simulink model "TEST_IPM_2_0"  (R2019b)
settings: configuration reference "Configuration" (kept outside this file)
PreLoadFcn:
  | RTWConfigurationCB('preloadfcn', bdroot);
values from neighbouring files (symbols this model uses):
  MParamFbase = 200.0    [TEST_IPM_LIB.sldd]
  MParamIbase = 360.0    [TEST_IPM_LIB.sldd]
  MParamLd = 8.0E-5    [TEST_IPM_LIB.sldd]
  MParamLq = 0.00028    [TEST_IPM_LIB.sldd]
  MParamRs = 0.014    [TEST_IPM_LIB.sldd]
  PWM_TPBRD_HALF = 5000.0    [TEST_IPM_LIB.sldd]
  Ts_10kHz = 0.0001    [TEST_IPM_LIB.sldd]
  Ts_1kHz = 0.001    [TEST_IPM_LIB.sldd]
undefined symbols (not defined in the file or in its folder): DiscIntNeverNeededParam, Down, GPTRIP1SEL, GPTRIP2SEL, TZ1, TZ2, Up
libraries: c280xlib x24, c2837xDlib x18, dsparch4 x11, c2802xlib x10, powerlib_meascontrol x9, dspstat3 x2, c2000lib x1, c2806xlib x1, idelinklib_common x1
(part 3 of 6)

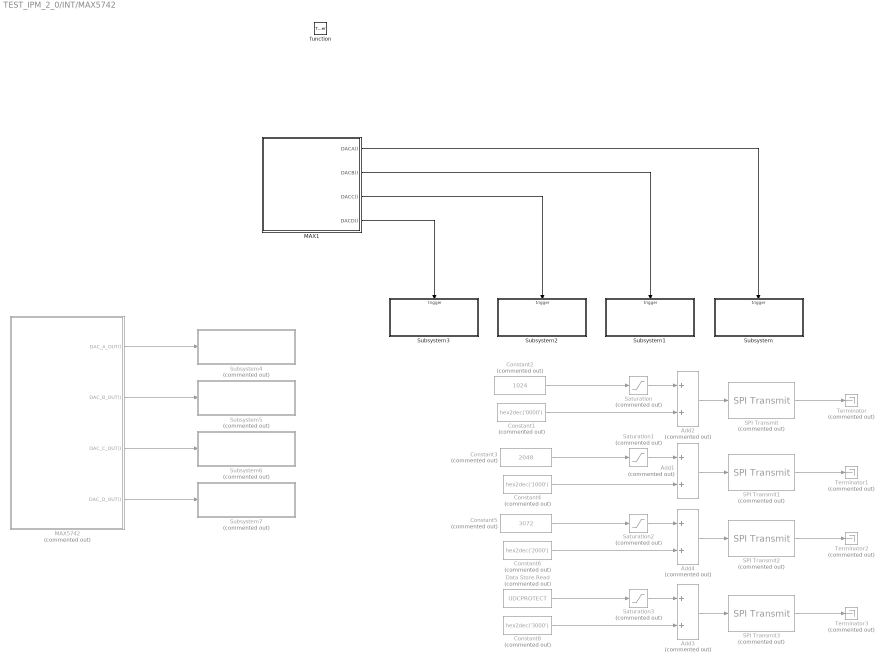
== system TEST_IPM_2_0/INT/MAX5742 ==
  function : TriggerPort  TriggerType=function-call  VariantControl=Variant
  Add{1..4} (4 alike) : Sum  Commented=on
  Constant1 : Constant  Commented=on  Value=hex2dec('0000')  OutDataTypeStr=uint16  SampleTime=-1
  Constant2 : Constant  Priority=102  Commented=on  Value=1024  OutDataTypeStr=Inherit: Inherit via back propagation  SampleTime=-1
  Constant3 : Constant  Priority=107  Commented=on  Value=2048  OutDataTypeStr=Inherit: Inherit via back propagation  SampleTime=-1
  Constant4 : Constant  Commented=on  Value=hex2dec('1000')  OutDataTypeStr=uint16  SampleTime=-1
  Constant5 : Constant  Priority=112  Commented=on  Value=3072  OutDataTypeStr=Inherit: Inherit via back propagation  SampleTime=-1
  Constant6 : Constant  Commented=on  Value=hex2dec('2000')  OutDataTypeStr=uint16  SampleTime=-1
  Constant8 : Constant  Commented=on  Value=hex2dec('3000')  OutDataTypeStr=uint16  SampleTime=-1
  Data Store Read : DataStoreRead  Commented=on  DataStoreName=UDCPROTECT
  MAX1 : MATLAB Function  TreatAsAtomicUnit=on
  MAX5742 : Stateflow chart  Commented=on  BlockKeywords=__PRM__SERIALIZED__DATA__:Stateflow Chart,Stateflow Diagram  TreatAsAtomicUnit=on
  SPI Transmit : c280xlib/SPI Transmit  Commented=on  SPISelect=SPI_B  ClockPolarity=Falling_edge  ClockPhase=No_delay  SPIModule=uint32(0)  Mode=Master  BusSpeed=uint32(1000000)  FirstBitToTransfer=Most significant bit (MSB)  ClockMode=0  BlockFunction=Write  EnableRegisterAddress=on  RegisterAddress=0  OutputDataType=int8  OutputDataLength=1  BlockingMode=off  DataBits=16  UseCustomSSPin=Provided by the SPI peripheral  ActiveLowSSPin=Active low  Pin=0
      settings: SourceProductName=Embedded Coder Support Package for Texas Instruments C2000 Processors  SourceProductBaseCode=TIC2000
  SPI Transmit1 : c280xlib/SPI Transmit  Commented=on  SPISelect=SPI_B  ClockPolarity=Rising_edge  ClockPhase=No_delay  SPIModule=uint32(0)  Mode=Master  BusSpeed=uint32(1000000)  FirstBitToTransfer=Most significant bit (MSB)  ClockMode=0  BlockFunction=Write  EnableRegisterAddress=on  RegisterAddress=0  OutputDataType=int8  OutputDataLength=1  BlockingMode=off  DataBits=16  UseCustomSSPin=Provided by the SPI peripheral  ActiveLowSSPin=Active low  Pin=0
      settings: SourceProductName=Embedded Coder Support Package for Texas Instruments C2000 Processors  SourceProductBaseCode=TIC2000
  SPI Transmit2 : c280xlib/SPI Transmit  Commented=on  SPISelect=SPI_B  ClockPolarity=Rising_edge  ClockPhase=No_delay  SPIModule=uint32(0)  Mode=Master  BusSpeed=uint32(1000000)  FirstBitToTransfer=Most significant bit (MSB)  ClockMode=0  BlockFunction=Write  EnableRegisterAddress=on  RegisterAddress=0  OutputDataType=int8  OutputDataLength=1  BlockingMode=off  DataBits=16  UseCustomSSPin=Provided by the SPI peripheral  ActiveLowSSPin=Active low  Pin=0
      settings: SourceProductName=Embedded Coder Support Package for Texas Instruments C2000 Processors  SourceProductBaseCode=TIC2000
  SPI Transmit3 : c280xlib/SPI Transmit  Commented=on  SPISelect=SPI_B  ClockPolarity=Rising_edge  ClockPhase=No_delay  SPIModule=uint32(0)  Mode=Master  BusSpeed=uint32(1000000)  FirstBitToTransfer=Most significant bit (MSB)  ClockMode=0  BlockFunction=Write  EnableRegisterAddress=on  RegisterAddress=0  OutputDataType=int8  OutputDataLength=1  BlockingMode=off  DataBits=16  UseCustomSSPin=Provided by the SPI peripheral  ActiveLowSSPin=Active low  Pin=0
      settings: SourceProductName=Embedded Coder Support Package for Texas Instruments C2000 Processors  SourceProductBaseCode=TIC2000
  Saturation{,1..3} (4 alike) : Saturate  Commented=on  UpperLimit=4095  LowerLimit=0  OutDataTypeStr=uint16
  Subsystem : Subsystem
  Subsystem1 : Subsystem
  Subsystem2 : Subsystem
  Subsystem3 : Subsystem
  Subsystem4 : Subsystem  Commented=on
  Subsystem5 : Subsystem  Commented=on
  Subsystem6 : Subsystem  Commented=on
  Subsystem7 : Subsystem  Commented=on
  Terminator{,1..3} (4 alike) : Terminator  Commented=on
  wires:
  MAX1/4(DACD()) -> Subsystem3/Trigger
  MAX1/3(DACC()) -> Subsystem2/Trigger
  MAX1/2(DACB()) -> Subsystem1/Trigger
  MAX1/1(DACA()) -> Subsystem/Trigger
  SPI Transmit/1 -> Terminator/1
  Add2/1 -> SPI Transmit/1
  Saturation/1 -> Add2/1
  Constant2/1 -> Saturation/1
  Constant1/1 -> Add2/2
  SPI Transmit1/1 -> Terminator1/1
  Constant4/1 -> Add1/2
  Add1/1 -> SPI Transmit1/1
  Saturation1/1 -> Add1/1
  Constant3/1 -> Saturation1/1
  Constant5/1 -> Saturation2/1
  Constant6/1 -> Add4/2
  Add4/1 -> SPI Transmit2/1
  Saturation2/1 -> Add4/1
  SPI Transmit2/1 -> Terminator2/1
  Saturation3/1 -> Add3/1
  Add3/1 -> SPI Transmit3/1
  SPI Transmit3/1 -> Terminator3/1
  Constant8/1 -> Add3/2
  Data Store Read/1 -> Saturation3/1
  MAX5742/1(DAC_A_OUT()) -> Subsystem4/Trigger
  MAX5742/2(DAC_B_OUT()) -> Subsystem5/Trigger
  MAX5742/3(DAC_C_OUT()) -> Subsystem6/Trigger
  MAX5742/4(DAC_D_OUT()) -> Subsystem7/Trigger

== system TEST_IPM_2_0/INT/Motor Control ==
  function : TriggerPort  TriggerType=function-call  VariantControl=Variant
  Adjusting Mode : Subsystem  TreatAsAtomicUnit=on
  Clark Transformation : Subsystem
  Current_PI : Subsystem  TreatAsAtomicUnit=on
      settings: RTWSystemCode=Inline
  Data Store Read1 : DataStoreRead  DataStoreName=ControlAng
  Data Store Read13 : DataStoreRead  DataStoreName=ControlAng
  Data Store Read14 : DataStoreRead  DataStoreName=Ud_in
  Data Store Read15 : DataStoreRead  DataStoreName=Uq_in
  Data Store Read16 : DataStoreRead  DataStoreName=W_Current
  Data Store Read2 : DataStoreRead  DataStoreName=ControlMode
  Data Store Read5 : DataStoreRead  DataStoreName=U_Current
  Data Store Read6 : DataStoreRead  DataStoreName=V_Current
  Data Store Write : DataStoreWrite  DataStoreName=COMPARE_A
  Data Store Write1 : DataStoreWrite  DataStoreName=COMPARE_B
  Data Store Write2 : DataStoreWrite  DataStoreName=COMPARE_C
  Data Store Write6 : DataStoreWrite  DataStoreName=Iq_FBK
  Data Store Write8 : DataStoreWrite  DataStoreName=Id_FBK
  Demux : Demux  Outputs=3
  Error : Subsystem  TreatAsAtomicUnit=on
  FbLMode : Subsystem  TreatAsAtomicUnit=on
  IF : Subsystem  TreatAsAtomicUnit=on
  Park Transformation : Subsystem
  SVPWM : Subsystem  TreatAsAtomicUnit=on
      settings: RTWSystemCode=Inline
  SpeedMode : Subsystem  TreatAsAtomicUnit=on
  "Stop " : Subsystem  TreatAsAtomicUnit=on
  Switch Case : SwitchCase  CaseConditions={0,1,2,3,4,5,6}
  TorqueMode : Subsystem  TreatAsAtomicUnit=on
  VF : Subsystem  TreatAsAtomicUnit=on
  wires:
  Data Store Read2/1 -> Switch Case/1
  Switch Case/1 -> Adjusting Mode/Action
  Switch Case/6 -> "Stop "/Action
  Switch Case/8 -> Error/Action
  Switch Case/2 -> VF/Action
  Switch Case/3 -> IF/Action
  Switch Case/4 -> TorqueMode/Action
  Switch Case/5 -> SpeedMode/Action
  Data Store Read1/1 -> SVPWM/3(Angle)
  Current_PI/1(Ud_Reference) -> SVPWM/1(Ud_Reference)
  Current_PI/2(Uq_Reference) -> SVPWM/2(Uq_Reference)
  SVPWM/1(COMPARE) -> Demux/1
  Demux/1 -> Data Store Write/1
  Demux/2 -> Data Store Write1/1
  Demux/3 -> Data Store Write2/1
  Data Store Read14/1 -> Current_PI/1(Ud)
  Data Store Read15/1 -> Current_PI/2(Uq)
  Switch Case/7 -> FbLMode/Action
  Data Store Read6/1 -> Clark Transformation/2(V)
  Data Store Read13/1 -> Park Transformation/3(theta)
  Clark Transformation/1(Alpha) -> Park Transformation/1(Alpha)
  Data Store Read16/1 -> Clark Transformation/3(W)
  Data Store Read5/1 -> Clark Transformation/1(U)
  Park Transformation/2(Q) -> Data Store Write6/1
  Park Transformation/1(D) -> Data Store Write8/1
  Clark Transformation/2(Beta) -> Park Transformation/2(Beta)

== system TEST_IPM_2_0/INT/Read Rotor Position ==
  function : TriggerPort  TriggerType=function-call  VariantControl=Variant
  Data Store Read : DataStoreRead  Priority=3  DataStoreName=SPIC_Tx
  Data Store Read1 : DataStoreRead  Priority=5  DataStoreName=SPIC_Tx
  Data Store Read3 : DataStoreRead  DataStoreName=ResloverMid
  Data Store Write : DataStoreWrite  DataStoreName=ResloverAng
  Data Store Write1 : DataStoreWrite  DataStoreName=SPIC_Rx
  Data Store Write14 : DataStoreWrite  DataStoreName=THERMAL_N
  Data Store Write2 : DataStoreWrite  DataStoreName=N_FBK
  Data Store Write3 : DataStoreWrite  DataStoreName=ResloverFaultRead
  Digital Output1 : c2837xDlib/Digital Output  GPIO_Number=GPIO48~GPIO55  GPIO_Bit0=off  GPIO_BIT0_Toggle=off  GPIO_Bit1=off  GPIO_BIT1_Toggle=off  GPIO_Bit2=off  GPIO_BIT2_Toggle=off  GPIO_Bit3=off  GPIO_BIT3_Toggle=off  GPIO_Bit4=off  GPIO_BIT4_Toggle=off  GPIO_Bit5=on  GPIO_BIT5_Toggle=off  GPIO_Bit6=off  GPIO_BIT6_Toggle=off  GPIO_Bit7=off  GPIO_BIT7_Toggle=off
      settings: SourceProductName=Embedded Coder Support Package for Texas Instruments C2000 Processors  SourceProductBaseCode=TIC2000
  Digital Output2 : c2837xDlib/Digital Output  GPIO_Number=GPIO48~GPIO55  GPIO_Bit0=off  GPIO_BIT0_Toggle=off  GPIO_Bit1=off  GPIO_BIT1_Toggle=off  GPIO_Bit2=off  GPIO_BIT2_Toggle=off  GPIO_Bit3=off  GPIO_BIT3_Toggle=off  GPIO_Bit4=off  GPIO_BIT4_Toggle=off  GPIO_Bit5=off  GPIO_BIT5_Toggle=off  GPIO_Bit6=on  GPIO_BIT6_Toggle=off  GPIO_Bit7=off  GPIO_BIT7_Toggle=off
      settings: SourceProductName=Embedded Coder Support Package for Texas Instruments C2000 Processors  SourceProductBaseCode=TIC2000
  Gain : Gain  Gain=2*pi
  MATLAB Function : MATLAB Function  TreatAsAtomicUnit=on
  "RAW_DATA2Angle " : MATLAB Function  TreatAsAtomicUnit=on
  ResloverWR1 : Constant  Priority=6  OutDataTypeStr=Inherit: Inherit via back propagation  SampleTime=-1
  ResloverWR2 : Constant  Priority=6  OutDataTypeStr=Inherit: Inherit via back propagation  SampleTime=-1
  SPI Master Transfer : c280xlib/SPI Master Transfer  SPISelect=SPI_C  ClockPolarity=Rising_edge  ClockPhase=No_delay  SPIModule=uint32(0)  Mode=Master  BusSpeed=uint32(1000000)  FirstBitToTransfer=Most significant bit (MSB)  ClockMode=0  BlockFunction=Transfer  EnableRegisterAddress=off  RegisterAddress=0  OutputDataType=int8  OutputDataLength=1  DataBits=16  UseCustomSSPin=Provided by the SPI peripheral  ActiveLowSSPin=Active low  Pin=1
      settings: SourceProductName=Embedded Coder Support Package for Texas Instruments C2000 Processors  SourceProductBaseCode=TIC2000
  SPI Master Transfer1 : c280xlib/SPI Master Transfer  SPISelect=SPI_C  ClockPolarity=Rising_edge  ClockPhase=No_delay  SPIModule=uint32(0)  Mode=Master  BusSpeed=uint32(1000000)  FirstBitToTransfer=Most significant bit (MSB)  ClockMode=0  BlockFunction=Transfer  EnableRegisterAddress=off  RegisterAddress=0  OutputDataType=int8  OutputDataLength=1  DataBits=8  UseCustomSSPin=Provided by the SPI peripheral  ActiveLowSSPin=Active low  Pin=1
      settings: SourceProductName=Embedded Coder Support Package for Texas Instruments C2000 Processors  SourceProductBaseCode=TIC2000
  SpeedCal : Subsystem  TreatAsAtomicUnit=on
  wires:
  Data Store Read/1 -> SPI Master Transfer/1
  SPI Master Transfer/1 -> "RAW_DATA2Angle "/1(Raw_Data), Data Store Write1/1
  ResloverWR1/1 -> Digital Output1/1
  Data Store Read3/1 -> "RAW_DATA2Angle "/2(Mid_Position)
  "RAW_DATA2Angle "/1(Angle_out) -> Gain/1
  SpeedCal/1(Out1) -> Data Store Write14/1, Data Store Write2/1
  MATLAB Function/1(FunCall()) -> SpeedCal/Trigger
  Data Store Read1/1 -> SPI Master Transfer1/1
  SPI Master Transfer1/1 -> Data Store Write3/1
  ResloverWR2/1 -> Digital Output2/1
  Gain/1 -> SpeedCal/1(In1), Data Store Write/1

== system TEST_IPM_2_0/INT/ePWM ==
  function : TriggerPort  TriggerType=function-call  VariantControl=Variant
  Constant2 : Constant  Value=[0 0]  OutDataTypeStr=uint16  SampleTime=-1
  Constant3 : Constant  Value=[1 2]  OutDataTypeStr=uint16  SampleTime=-1
  Data Store Read1 : DataStoreRead  DataStoreName=STOP
  Data Store Read3 : DataStoreRead  DataStoreName=COMPARE_A
  Data Store Read4 : DataStoreRead  DataStoreName=COMPARE_B
  Data Store Read7 : DataStoreRead  DataStoreName=COMPARE_C
  Demux : Demux  Outputs=2
  If : If  IfExpression=u1 == 1
  If Action Subsystem : Subsystem  TreatAsAtomicUnit=on
  Switch : Switch  Criteria=u2 ~= 0
  ePWM : c2802xlib/ePWM  useModule=ePWM1  ePWMxLINKTBPRD=Not Linked  periodUnits=Clock cycles  timerSource=Specify via dialog  timerPeriod_clk=PWM_TPBRD  timerPeriod_sec=Tsw  tbshadow=Counter equals to zero  countingMode=Up-Down  phaseActiveEnable=Disable  phaseDirection=Count down after sync  phaseActive=0  synchronizationEnable=off  dcaevt1Sync=off  dcbevt1Sync=off  synchronizationOption=Counter equals to zero (CTR=Zero)  clockPrescale=1  HSclockPrescale=1  enswap=off  ePWMxAStatus=on  ePWMxAactionLogic1=Do nothing  ePWMxAactionLogic2=Do nothing  ePWMxAactionLogic3=Clear  ePWMxAactionLogic4=Set  ePWMxAactionLogic5=Do nothing  ePWMxAactionLogic6=Do nothing  ePWMxALoadMode=Load on counter equals to zero (CTR=Zero)  ePWMxACSFenable=on  ePWMxACSFvalue=Forcing disable  ePWMxASFreload=Immediate  ePWMxBStatus=on  ePWMxBactionLogic1=Do nothing  ePWMxBactionLogic2=Do nothing  ePWMxBactionLogic3=Clear  ePWMxBactionLogic4=Set  ePWMxBactionLogic5=Do nothing  ePWMxBactionLogic6=Do nothing  ePWMxBLoadMode=Load on counter equals to zero (CTR=Zero)  ePWMxBCSFenable=on  ePWMxBCSFvalue=Forcing disable  ePWMxBSFreload=Immediate  ePWNxBOutWay=off  ePWMxLINKCMPA=Not Linked  CMPAUnits=Clock cycles  CMPASource=Input port  CMPAValue_per=50  CMPAValue_clk=PWM_TPBRD_HALF  enCMPAshadow=Counter equals to zero  ePWMxLINKCMPB=Not Linked  CMPBUnits=Percentages  CMPBSource=Specify via dialog  CMPBValue_per=50  CMPBValue_clk=32000  enCMPBshadow=Counter equals to zero  ePWMxLINKCMPC=Not Linked  CMPCUnits=Clock cycles  CMPCSource=Specify via dialog  CMPCValue_per=50  CMPCValue_clk=32000  enCMPCshadow=Counter equals to zero  ePWMxLINKCMPD=Not Linked  CMPDUnits=Clock cycles  CMPDSource=Specify via dialog  CMPDValue_per=50  CMPDValue_clk=32000  enCMPDshadow=Counter equals to zero  enableDBePWMxA=on  enableDBePWMxB=on  enhalfcycle=off  DBpolarity=Active high complementary (AHC)  DBedgeDelay=Positive  DBSource_ePWMxA=ePWMxA  DBSource_ePWMxB=ePWMxB  DBperiodSource=Specify via dialog  REDperiod=PWM_TDEAD  FEDperiod=PWM_TDEAD  adcstartModuleA=on  adcrequestEventA=First event  adcstartEventA=Digital Compare Module A Event 1 start of conversion (DCAEVT1.soc)  adcstartEventA_type2=Counter equals to zero (CTR=Zero)  adcstartModuleB=off  adcrequestEventB=First event  adcstartEventB=Counter equals to zero (CTR=Zero)  adcstartEventB_type2=Counter equals to zero (CTR=Zero)  intEn=off  intPrd=First event  intSel=Counter equals to zero (CTR=Zero)  intSel_type2=Counter equals to period (CTR=PRD)  hrpe=off  enHRPWM=off  HRPWM_LoadMode=Counter equals to period (CTR=PRD)  HRPWM_CTLMode=Duty or Period control mode  HRPWM_EDGMode=Both edge  hrpeb=off  enHRPWMB=off  HRPWM_LoadModeB=Counter equals to zero (CTR=ZERO)  HRPWM_CTLModeB=Duty or Period control mode  HRPWM_EDGModeB=Both edge  enSFO=on  enautoconv=on  chopperEnable=off  chopperFrequency=1  chopperFirstwidth=1  chopperDuty=12.5%  tripZonesource=Specify via dialog  tzselOSHT1=off  tzselOSHT2=off  tzselOSHT3=off  tzselOSHDCAEV1=off  tzselOSHDCBEV1=off  tzselCBC1=off  tzselCBC2=off  tzselCBC3=off  tzselCBCDCAEV2=off  tzselCBCDCBEV2=off  tzselOSHT4=off  tzselOSHT5=off  tzselOSHT6=off  tzselCBC4=off  tzselCBC5=off  tzselCBC6=off  enTzOstIntr=on  enTzCbcIntr=off  enTzDCAEVT1Intr=off  enTzDCAEVT2Intr=off  enTzDCBEVT1Intr=off  enTzDCBEVT2Intr=off  ePWMxAforced=Low  ePWMxBforced=Low  DCAEVT1forced=No action  DCBEVT1forced=No action  DCAEVT2forced=No action  DCBEVT2forced=No action  dcah=Trip Zone 1 input (TZ1)  dcal=Trip Zone 2 input (TZ2)  dcbh=Trip Zone 1 input (TZ1)  dcbl=Trip Zone 2 input (TZ2)  dcah_type2=GPTRIP1SEL/(TZ1)  dcal_type2=GPTRIP2SEL/(TZ2)  dcbh_type2=GPTRIP1SEL/(TZ1)  dcbl_type2=GPTRIP2SEL/(TZ2)  gendcaevt1=Event disabled  gendcaevt2=Event disabled  gendcbevt1=Event disabled  gendcbevt2=Event disabled  dcaevt1src=DCAEVT1 with sync  dcaevt2src=DCAEVT2 with sync  dcbevt1src=DCBEVT1 with sync  dcbevt2src=DCBEVT2 with sync  pulsesel=Counter equals to zero (CTR=Zero)  blankinv=off  blankoffset=0  blankwidth=0  evsrcsel=Filtered version of DCAEVT1 (DCAEVT1FILT)  encape=off  PwmType=C2000_Type4
      settings: SourceProductName=Embedded Coder Support Package for Texas Instruments C2000 Processors
  ePWM1 : c2802xlib/ePWM  useModule=ePWM2  ePWMxLINKTBPRD=Not Linked  periodUnits=Clock cycles  timerSource=Specify via dialog  timerPeriod_clk=PWM_TPBRD  timerPeriod_sec=Tsw  tbshadow=Counter equals to zero  countingMode=Up-Down  phaseActiveEnable=Set counter to phase value specified via dialog  phaseDirection=Count down after sync  phaseActive=0  synchronizationEnable=off  dcaevt1Sync=off  dcbevt1Sync=off  synchronizationOption=Disable  clockPrescale=1  HSclockPrescale=1  enswap=off  ePWMxAStatus=on  ePWMxAactionLogic1=Do nothing  ePWMxAactionLogic2=Do nothing  ePWMxAactionLogic3=Clear  ePWMxAactionLogic4=Set  ePWMxAactionLogic5=Do nothing  ePWMxAactionLogic6=Do nothing  ePWMxALoadMode=Load on counter equals to zero (CTR=Zero)  ePWMxACSFenable=on  ePWMxACSFvalue=Forcing disable  ePWMxASFreload=Immediate  ePWMxBStatus=on  ePWMxBactionLogic1=Do nothing  ePWMxBactionLogic2=Do nothing  ePWMxBactionLogic3=Clear  ePWMxBactionLogic4=Set  ePWMxBactionLogic5=Do nothing  ePWMxBactionLogic6=Do nothing  ePWMxBLoadMode=Load on counter equals to zero (CTR=Zero)  ePWMxBCSFenable=on  ePWMxBCSFvalue=Forcing disable  ePWMxBSFreload=Immediate  ePWNxBOutWay=off  ePWMxLINKCMPA=Not Linked  CMPAUnits=Clock cycles  CMPASource=Input port  CMPAValue_per=50  CMPAValue_clk=PWM_TPBRD_HALF  enCMPAshadow=Counter equals to zero  ePWMxLINKCMPB=Not Linked  CMPBUnits=Percentages  CMPBSource=Specify via dialog  CMPBValue_per=50  CMPBValue_clk=32000  enCMPBshadow=Counter equals to zero  ePWMxLINKCMPC=Not Linked  CMPCUnits=Clock cycles  CMPCSource=Specify via dialog  CMPCValue_per=50  CMPCValue_clk=32000  enCMPCshadow=Counter equals to zero  ePWMxLINKCMPD=Not Linked  CMPDUnits=Clock cycles  CMPDSource=Specify via dialog  CMPDValue_per=50  CMPDValue_clk=32000  enCMPDshadow=Counter equals to zero  enableDBePWMxA=on  enableDBePWMxB=on  enhalfcycle=off  DBpolarity=Active high complementary (AHC)  DBedgeDelay=Positive  DBSource_ePWMxA=ePWMxA  DBSource_ePWMxB=ePWMxB  DBperiodSource=Specify via dialog  REDperiod=PWM_TDEAD  FEDperiod=PWM_TDEAD  adcstartModuleA=off  adcrequestEventA=First event  adcstartEventA=Digital Compare Module A Event 1 start of conversion (DCAEVT1.soc)  adcstartEventA_type2=Counter equals to period (CTR=PRD)  adcstartModuleB=off  adcrequestEventB=First event  adcstartEventB=Counter equals to zero (CTR=Zero)  adcstartEventB_type2=Counter equals to zero (CTR=Zero)  intEn=off  intPrd=First event  intSel=Counter equals to zero (CTR=Zero)  intSel_type2=Counter equals to period (CTR=PRD)  hrpe=off  enHRPWM=off  HRPWM_LoadMode=Counter equals to period (CTR=PRD)  HRPWM_CTLMode=Duty or Period control mode  HRPWM_EDGMode=Both edge  hrpeb=off  enHRPWMB=off  HRPWM_LoadModeB=Counter equals to zero (CTR=ZERO)  HRPWM_CTLModeB=Duty or Period control mode  HRPWM_EDGModeB=Both edge  enSFO=on  enautoconv=on  chopperEnable=off  chopperFrequency=1  chopperFirstwidth=1  chopperDuty=12.5%  tripZonesource=Specify via dialog  tzselOSHT1=off  tzselOSHT2=off  tzselOSHT3=off  tzselOSHDCAEV1=off  tzselOSHDCBEV1=off  tzselCBC1=off  tzselCBC2=off  tzselCBC3=off  tzselCBCDCAEV2=off  tzselCBCDCBEV2=off  tzselOSHT4=off  tzselOSHT5=off  tzselOSHT6=off  tzselCBC4=off  tzselCBC5=off  tzselCBC6=off  enTzOstIntr=on  enTzCbcIntr=off  enTzDCAEVT1Intr=off  enTzDCAEVT2Intr=off  enTzDCBEVT1Intr=off  enTzDCBEVT2Intr=off  ePWMxAforced=Low  ePWMxBforced=Low  DCAEVT1forced=No action  DCBEVT1forced=No action  DCAEVT2forced=No action  DCBEVT2forced=No action  dcah=Trip Zone 1 input (TZ1)  dcal=Trip Zone 2 input (TZ2)  dcbh=Trip Zone 1 input (TZ1)  dcbl=Trip Zone 2 input (TZ2)  dcah_type2=GPTRIP1SEL/(TZ1)  dcal_type2=GPTRIP2SEL/(TZ2)  dcbh_type2=GPTRIP1SEL/(TZ1)  dcbl_type2=GPTRIP2SEL/(TZ2)  gendcaevt1=Event disabled  gendcaevt2=Event disabled  gendcbevt1=Event disabled  gendcbevt2=Event disabled  dcaevt1src=DCAEVT1 with sync  dcaevt2src=DCAEVT2 with sync  dcbevt1src=DCBEVT1 with sync  dcbevt2src=DCBEVT2 with sync  pulsesel=Counter equals to zero (CTR=Zero)  blankinv=off  blankoffset=0  blankwidth=0  evsrcsel=Filtered version of DCAEVT1 (DCAEVT1FILT)  encape=off  PwmType=C2000_Type4
      settings: SourceProductName=Embedded Coder Support Package for Texas Instruments C2000 Processors
  ePWM2 : c2802xlib/ePWM  useModule=ePWM3  ePWMxLINKTBPRD=Not Linked  periodUnits=Clock cycles  timerSource=Specify via dialog  timerPeriod_clk=PWM_TPBRD  timerPeriod_sec=Tsw  tbshadow=Counter equals to zero  countingMode=Up-Down  phaseActiveEnable=Set counter to phase value specified via dialog  phaseDirection=Count down after sync  phaseActive=0  synchronizationEnable=off  dcaevt1Sync=off  dcbevt1Sync=off  synchronizationOption=Disable  clockPrescale=1  HSclockPrescale=1  enswap=off  ePWMxAStatus=on  ePWMxAactionLogic1=Do nothing  ePWMxAactionLogic2=Do nothing  ePWMxAactionLogic3=Clear  ePWMxAactionLogic4=Set  ePWMxAactionLogic5=Do nothing  ePWMxAactionLogic6=Do nothing  ePWMxALoadMode=Load on counter equals to zero (CTR=Zero)  ePWMxACSFenable=on  ePWMxACSFvalue=Forcing disable  ePWMxASFreload=Immediate  ePWMxBStatus=on  ePWMxBactionLogic1=Do nothing  ePWMxBactionLogic2=Do nothing  ePWMxBactionLogic3=Clear  ePWMxBactionLogic4=Set  ePWMxBactionLogic5=Do nothing  ePWMxBactionLogic6=Do nothing  ePWMxBLoadMode=Load on counter equals to zero (CTR=Zero)  ePWMxBCSFenable=on  ePWMxBCSFvalue=Forcing disable  ePWMxBSFreload=Immediate  ePWNxBOutWay=off  ePWMxLINKCMPA=Not Linked  CMPAUnits=Clock cycles  CMPASource=Input port  CMPAValue_per=50  CMPAValue_clk=PWM_TPBRD_HALF  enCMPAshadow=Counter equals to zero  ePWMxLINKCMPB=Not Linked  CMPBUnits=Percentages  CMPBSource=Specify via dialog  CMPBValue_per=50  CMPBValue_clk=32000  enCMPBshadow=Counter equals to zero  ePWMxLINKCMPC=Not Linked  CMPCUnits=Clock cycles  CMPCSource=Specify via dialog  CMPCValue_per=50  CMPCValue_clk=32000  enCMPCshadow=Counter equals to zero  ePWMxLINKCMPD=Not Linked  CMPDUnits=Clock cycles  CMPDSource=Specify via dialog  CMPDValue_per=50  CMPDValue_clk=32000  enCMPDshadow=Counter equals to zero  enableDBePWMxA=on  enableDBePWMxB=on  enhalfcycle=off  DBpolarity=Active high complementary (AHC)  DBedgeDelay=Positive  DBSource_ePWMxA=ePWMxA  DBSource_ePWMxB=ePWMxB  DBperiodSource=Specify via dialog  REDperiod=PWM_TDEAD  FEDperiod=PWM_TDEAD  adcstartModuleA=off  adcrequestEventA=First event  adcstartEventA=Digital Compare Module A Event 1 start of conversion (DCAEVT1.soc)  adcstartEventA_type2=Counter equals to zero (CTR=Zero)  adcstartModuleB=off  adcrequestEventB=First event  adcstartEventB=Counter equals to zero (CTR=Zero)  adcstartEventB_type2=Counter equals to zero (CTR=Zero)  intEn=off  intPrd=First event  intSel=Counter equals to zero (CTR=Zero)  intSel_type2=Counter equals to period (CTR=PRD)  hrpe=off  enHRPWM=off  HRPWM_LoadMode=Counter equals to period (CTR=PRD)  HRPWM_CTLMode=Duty or Period control mode  HRPWM_EDGMode=Both edge  hrpeb=off  enHRPWMB=off  HRPWM_LoadModeB=Counter equals to zero (CTR=ZERO)  HRPWM_CTLModeB=Duty or Period control mode  HRPWM_EDGModeB=Both edge  enSFO=on  enautoconv=on  chopperEnable=off  chopperFrequency=1  chopperFirstwidth=1  chopperDuty=12.5%  tripZonesource=Specify via dialog  tzselOSHT1=off  tzselOSHT2=off  tzselOSHT3=off  tzselOSHDCAEV1=off  tzselOSHDCBEV1=off  tzselCBC1=off  tzselCBC2=off  tzselCBC3=off  tzselCBCDCAEV2=off  tzselCBCDCBEV2=off  tzselOSHT4=off  tzselOSHT5=off  tzselOSHT6=off  tzselCBC4=off  tzselCBC5=off  tzselCBC6=off  enTzOstIntr=on  enTzCbcIntr=off  enTzDCAEVT1Intr=off  enTzDCAEVT2Intr=off  enTzDCBEVT1Intr=off  enTzDCBEVT2Intr=off  ePWMxAforced=Low  ePWMxBforced=Low  DCAEVT1forced=No action  DCBEVT1forced=No action  DCAEVT2forced=No action  DCBEVT2forced=No action  dcah=Trip Zone 1 input (TZ1)  dcal=Trip Zone 2 input (TZ2)  dcbh=Trip Zone 1 input (TZ1)  dcbl=Trip Zone 2 input (TZ2)  dcah_type2=GPTRIP1SEL/(TZ1)  dcal_type2=GPTRIP2SEL/(TZ2)  dcbh_type2=GPTRIP1SEL/(TZ1)  dcbl_type2=GPTRIP2SEL/(TZ2)  gendcaevt1=Event disabled  gendcaevt2=Event disabled  gendcbevt1=Event disabled  gendcbevt2=Event disabled  dcaevt1src=DCAEVT1 with sync  dcaevt2src=DCAEVT2 with sync  dcbevt1src=DCBEVT1 with sync  dcbevt2src=DCBEVT2 with sync  pulsesel=Counter equals to zero (CTR=Zero)  blankinv=off  blankoffset=0  blankwidth=0  evsrcsel=Filtered version of DCAEVT1 (DCAEVT1FILT)  encape=off  PwmType=C2000_Type4
      settings: SourceProductName=Embedded Coder Support Package for Texas Instruments C2000 Processors
  wires:
  Constant3/1 -> Switch/1
  Constant2/1 -> Switch/3
  Demux/2 -> ePWM1/3, ePWM/3, ePWM2/3
  Data Store Read1/1 -> If/1, Switch/2
  Switch/1 -> Demux/1
  Demux/1 -> ePWM2/2, ePWM1/2, ePWM/2
  Data Store Read7/1 -> ePWM2/1
  Data Store Read3/1 -> ePWM/1
  Data Store Read4/1 -> ePWM1/1
  If/1 -> If Action Subsystem/Action

== system TEST_IPM_2_0/SpeedREF/Subsystem1 ==
  TargetValue : Inport
  Step : Inport  Port=2
  MATLAB Function : MATLAB Function  TreatAsAtomicUnit=on
  Unit Delay : UnitDelay  SampleTime=-1  HasFrameUpgradeWarning=on
  RampOutput : Outport
  wires:
  TargetValue/1 -> MATLAB Function/1(Target)
  MATLAB Function/1(Output) -> RampOutput/1, Unit Delay/1
  Step/1 -> MATLAB Function/2(Step)
  Unit Delay/1 -> MATLAB Function/3(LastOutput)

== system TEST_IPM_2_0/Temperature&DCBUS/Function-Call Subsystem ==
  function : TriggerPort  TriggerType=function-call  VariantControl=Variant
  Constant : Constant  Priority=0  Value=0  SampleTime=-1
  Digital Output : c2837xDlib/Digital Output  GPIO_Number=GPIO112~GPIO119  GPIO_Bit0=off  GPIO_BIT0_Toggle=off  GPIO_Bit1=on  GPIO_BIT1_Toggle=off  GPIO_Bit2=off  GPIO_BIT2_Toggle=off  GPIO_Bit3=off  GPIO_BIT3_Toggle=off  GPIO_Bit4=off  GPIO_BIT4_Toggle=off  GPIO_Bit5=off  GPIO_BIT5_Toggle=off  GPIO_Bit6=off  GPIO_BIT6_Toggle=off  GPIO_Bit7=off  GPIO_BIT7_Toggle=off
      settings: SourceProductName=Embedded Coder Support Package for Texas Instruments C2000 Processors  SourceProductBaseCode=TIC2000
  wires:
  Constant/1 -> Digital Output/1

== system TEST_IPM_2_0/Temperature&DCBUS/Function-Call Subsystem1 ==
  function : TriggerPort  TriggerType=function-call  VariantControl=Variant
  Constant1 : Constant  Value=10  OutDataTypeStr=single  SampleTime=-1
  Constant2 : Constant  Priority=2  Value=20  OutDataTypeStr=single  SampleTime=-1
  Constant4 : Constant  OutDataTypeStr=single  SampleTime=-1
  Data Store Read2 : DataStoreRead  DataStoreName=DEKF_Rs
  Data Store Read3 : DataStoreRead  DataStoreName=DEKF_Ldd
  Data Store Read7 : DataStoreRead  DataStoreName=DEKF_Ldq
  Data Store Write10 : DataStoreWrite  DataStoreName=DEKF_Lqq
  Data Store Write7 : DataStoreWrite  DataStoreName=DEKF_Rs
  Data Store Write8 : DataStoreWrite  DataStoreName=DEKF_Ldd
  Data Store Write9 : DataStoreWrite  DataStoreName=DEKF_Ldq
  MATLAB Function5 : MATLAB Function  TreatAsAtomicUnit=on
  Unit Delay{,1..4} (5 alike) : UnitDelay  InitialCondition=20  SampleTime=-1  HasFrameUpgradeWarning=on
  wires:
  MATLAB Function5/4(Tew_Calk1) -> Data Store Write10/1, Unit Delay1/1
  MATLAB Function5/2(Ts_Calk1) -> Data Store Write8/1, Unit Delay3/1
  Unit Delay3/1 -> MATLAB Function5/6(Ts_Calk0)
  Data Store Read7/1 -> MATLAB Function5/3(Speed_Sam)
  MATLAB Function5/6(Tem_Cal) -> ?
  Data Store Read3/1 -> MATLAB Function5/2(Iq_Sam)
  MATLAB Function5/1(Tr_Calk1) -> Data Store Write7/1, Unit Delay4/1
  MATLAB Function5/3(Tw_Calk1) -> Data Store Write9/1, Unit Delay2/1
  Unit Delay4/1 -> MATLAB Function5/5(Tr_Calk0)
  Unit Delay1/1 -> MATLAB Function5/8(Tew_Calk0)
  Constant2/1 -> MATLAB Function5/10(Tf_Sam)
  Unit Delay2/1 -> MATLAB Function5/7(Tw_Calk0)
  Constant1/1 -> MATLAB Function5/11(Flowrate)
  MATLAB Function5/5(Tb_Calk1) -> Unit Delay/1
  Data Store Read2/1 -> MATLAB Function5/1(Id_Sam)
  Unit Delay/1 -> MATLAB Function5/9(Tb_Calk0)
  Constant4/1 -> MATLAB Function5/4(Ts)

== system TEST_IPM_2_0/Temperature&DCBUS/Function-Call Subsystem2 ==
  function : TriggerPort  TriggerType=function-call  VariantControl=Variant
  Constant3 : Constant  Priority=10  OutDataTypeStr=uint16  SampleTime=-1
  Digital Output1 : c2837xDlib/Digital Output  GPIO_Number=GPIO112~GPIO119  GPIO_Bit0=off  GPIO_BIT0_Toggle=off  GPIO_Bit1=on  GPIO_BIT1_Toggle=off  GPIO_Bit2=off  GPIO_BIT2_Toggle=off  GPIO_Bit3=off  GPIO_BIT3_Toggle=off  GPIO_Bit4=off  GPIO_BIT4_Toggle=off  GPIO_Bit5=off  GPIO_BIT5_Toggle=off  GPIO_Bit6=off  GPIO_BIT6_Toggle=off  GPIO_Bit7=off  GPIO_BIT7_Toggle=off
      settings: SourceProductName=Embedded Coder Support Package for Texas Instruments C2000 Processors  SourceProductBaseCode=TIC2000
  wires:
  Constant3/1 -> Digital Output1/1

== system TEST_IPM_2_0/UdcREF/Subsystem1 ==
  TargetValue : Inport
  Step : Inport  Port=2
  MATLAB Function : MATLAB Function  TreatAsAtomicUnit=on
  Unit Delay : UnitDelay  SampleTime=-1  HasFrameUpgradeWarning=on
  RampOutput : Outport
  wires:
  Unit Delay/1 -> MATLAB Function/3(LastOutput)
  Step/1 -> MATLAB Function/2(Step)
  MATLAB Function/1(Output) -> Unit Delay/1, RampOutput/1
  TargetValue/1 -> MATLAB Function/1(Target)

== system TEST_IPM_2_0/INT/AD2S1210 Init/Function-Call Subsystem ==
  function : TriggerPort  TriggerType=function-call  VariantControl=Variant
  Data Store Read : DataStoreRead  DataStoreName=ResloverRESET
  Digital Output : c2837xDlib/Digital Output  GPIO_Number=GPIO48~GPIO55  GPIO_Bit0=off  GPIO_BIT0_Toggle=off  GPIO_Bit1=off  GPIO_BIT1_Toggle=off  GPIO_Bit2=off  GPIO_BIT2_Toggle=off  GPIO_Bit3=off  GPIO_BIT3_Toggle=off  GPIO_Bit4=off  GPIO_BIT4_Toggle=off  GPIO_Bit5=off  GPIO_BIT5_Toggle=off  GPIO_Bit6=off  GPIO_BIT6_Toggle=off  GPIO_Bit7=on  GPIO_BIT7_Toggle=off
      settings: SourceProductName=Embedded Coder Support Package for Texas Instruments C2000 Processors  SourceProductBaseCode=TIC2000
  wires:
  Data Store Read/1 -> Digital Output/1

== system TEST_IPM_2_0/INT/AD2S1210 Init/Function-Call Subsystem1 ==
  function : TriggerPort  TriggerType=function-call  VariantControl=Variant
  Data Store Read : DataStoreRead  DataStoreName=ResloverWR
  Digital Output : c2837xDlib/Digital Output  GPIO_Number=GPIO48~GPIO55  GPIO_Bit0=off  GPIO_BIT0_Toggle=off  GPIO_Bit1=off  GPIO_BIT1_Toggle=off  GPIO_Bit2=off  GPIO_BIT2_Toggle=off  GPIO_Bit3=off  GPIO_BIT3_Toggle=off  GPIO_Bit4=off  GPIO_BIT4_Toggle=off  GPIO_Bit5=on  GPIO_BIT5_Toggle=off  GPIO_Bit6=off  GPIO_BIT6_Toggle=off  GPIO_Bit7=off  GPIO_BIT7_Toggle=off
      settings: SourceProductName=Embedded Coder Support Package for Texas Instruments C2000 Processors  SourceProductBaseCode=TIC2000
  wires:
  Data Store Read/1 -> Digital Output/1

== system TEST_IPM_2_0/INT/AD2S1210 Init/Function-Call Subsystem2 ==
  function : TriggerPort  TriggerType=function-call  VariantControl=Variant
  Data Store Read : DataStoreRead  Priority=1  DataStoreName=ResloverWR
  Data Store Read1 : DataStoreRead  Priority=4  DataStoreName=SPIC_Tx
  Data Store Write : DataStoreWrite  DataStoreName=SPIC_Rx
  Digital Output : c2837xDlib/Digital Output  GPIO_Number=GPIO48~GPIO55  GPIO_Bit0=off  GPIO_BIT0_Toggle=off  GPIO_Bit1=off  GPIO_BIT1_Toggle=off  GPIO_Bit2=off  GPIO_BIT2_Toggle=off  GPIO_Bit3=off  GPIO_BIT3_Toggle=off  GPIO_Bit4=off  GPIO_BIT4_Toggle=off  GPIO_Bit5=on  GPIO_BIT5_Toggle=off  GPIO_Bit6=off  GPIO_BIT6_Toggle=off  GPIO_Bit7=off  GPIO_BIT7_Toggle=off
      settings: SourceProductName=Embedded Coder Support Package for Texas Instruments C2000 Processors  SourceProductBaseCode=TIC2000
  S-Function1 : S-Function  Priority=3  Commented=on  FunctionName=User_Defined_Code  Parameters=code  SFunctionDeploymentMode=off  EnableBusSupport=off  mask{code=DELAY_US(1u);}
  SPI Master Transfer : c280xlib/SPI Master Transfer  SPISelect=SPI_C  ClockPolarity=Rising_edge  ClockPhase=No_delay  SPIModule=uint32(0)  Mode=Master  BusSpeed=uint32(1000000)  FirstBitToTransfer=Most significant bit (MSB)  ClockMode=0  BlockFunction=Transfer  EnableRegisterAddress=off  RegisterAddress=0  OutputDataType=int8  OutputDataLength=1  DataBits=16  UseCustomSSPin=Provided by the SPI peripheral  ActiveLowSSPin=Active low  Pin=1
      settings: SourceProductName=Embedded Coder Support Package for Texas Instruments C2000 Processors  SourceProductBaseCode=TIC2000
  wires:
  Data Store Read1/1 -> SPI Master Transfer/1
  SPI Master Transfer/1 -> Data Store Write/1
  Data Store Read/1 -> Digital Output/1

== system TEST_IPM_2_0/INT/AD2S1210 Init/Function-Call Subsystem3 ==
  function : TriggerPort  TriggerType=function-call  VariantControl=Variant
  Data Store Read : DataStoreRead  DataStoreName=ResloverA0
  Data Store Read1 : DataStoreRead  DataStoreName=ResloverA1
  Digital Output : c2837xDlib/Digital Output  GPIO_Number=GPIO56~GPIO63  GPIO_Bit0=off  GPIO_BIT0_Toggle=off  GPIO_Bit1=off  GPIO_BIT1_Toggle=off  GPIO_Bit2=on  GPIO_BIT2_Toggle=off  GPIO_Bit3=off  GPIO_BIT3_Toggle=off  GPIO_Bit4=off  GPIO_BIT4_Toggle=off  GPIO_Bit5=off  GPIO_BIT5_Toggle=off  GPIO_Bit6=off  GPIO_BIT6_Toggle=off  GPIO_Bit7=off  GPIO_BIT7_Toggle=off
      settings: SourceProductName=Embedded Coder Support Package for Texas Instruments C2000 Processors  SourceProductBaseCode=TIC2000
  Digital Output1 : c2837xDlib/Digital Output  GPIO_Number=GPIO56~GPIO63  GPIO_Bit0=off  GPIO_BIT0_Toggle=off  GPIO_Bit1=off  GPIO_BIT1_Toggle=off  GPIO_Bit2=off  GPIO_BIT2_Toggle=off  GPIO_Bit3=on  GPIO_BIT3_Toggle=off  GPIO_Bit4=off  GPIO_BIT4_Toggle=off  GPIO_Bit5=off  GPIO_BIT5_Toggle=off  GPIO_Bit6=off  GPIO_BIT6_Toggle=off  GPIO_Bit7=off  GPIO_BIT7_Toggle=off
      settings: SourceProductName=Embedded Coder Support Package for Texas Instruments C2000 Processors  SourceProductBaseCode=TIC2000
  wires:
  Data Store Read/1 -> Digital Output/1
  Data Store Read1/1 -> Digital Output1/1

== system TEST_IPM_2_0/INT/AD2S1210 Init/Function-Call Subsystem4 ==
  function : TriggerPort  TriggerType=function-call  VariantControl=Variant
  Data Store Read : DataStoreRead  DataStoreName=ResloverA0
  Data Store Read1 : DataStoreRead  DataStoreName=ResloverA1
  Data Store Read2 : DataStoreRead  DataStoreName=ResloverWR
  Digital Output : c2837xDlib/Digital Output  GPIO_Number=GPIO56~GPIO63  GPIO_Bit0=off  GPIO_BIT0_Toggle=off  GPIO_Bit1=off  GPIO_BIT1_Toggle=off  GPIO_Bit2=on  GPIO_BIT2_Toggle=off  GPIO_Bit3=off  GPIO_BIT3_Toggle=off  GPIO_Bit4=off  GPIO_BIT4_Toggle=off  GPIO_Bit5=off  GPIO_BIT5_Toggle=off  GPIO_Bit6=off  GPIO_BIT6_Toggle=off  GPIO_Bit7=off  GPIO_BIT7_Toggle=off
      settings: SourceProductName=Embedded Coder Support Package for Texas Instruments C2000 Processors  SourceProductBaseCode=TIC2000
  Digital Output1 : c2837xDlib/Digital Output  GPIO_Number=GPIO56~GPIO63  GPIO_Bit0=off  GPIO_BIT0_Toggle=off  GPIO_Bit1=off  GPIO_BIT1_Toggle=off  GPIO_Bit2=off  GPIO_BIT2_Toggle=off  GPIO_Bit3=on  GPIO_BIT3_Toggle=off  GPIO_Bit4=off  GPIO_BIT4_Toggle=off  GPIO_Bit5=off  GPIO_BIT5_Toggle=off  GPIO_Bit6=off  GPIO_BIT6_Toggle=off  GPIO_Bit7=off  GPIO_BIT7_Toggle=off
      settings: SourceProductName=Embedded Coder Support Package for Texas Instruments C2000 Processors  SourceProductBaseCode=TIC2000
  Digital Output2 : c2837xDlib/Digital Output  GPIO_Number=GPIO48~GPIO55  GPIO_Bit0=off  GPIO_BIT0_Toggle=off  GPIO_Bit1=off  GPIO_BIT1_Toggle=off  GPIO_Bit2=off  GPIO_BIT2_Toggle=off  GPIO_Bit3=off  GPIO_BIT3_Toggle=off  GPIO_Bit4=off  GPIO_BIT4_Toggle=off  GPIO_Bit5=on  GPIO_BIT5_Toggle=off  GPIO_Bit6=off  GPIO_BIT6_Toggle=off  GPIO_Bit7=off  GPIO_BIT7_Toggle=off
      settings: SourceProductName=Embedded Coder Support Package for Texas Instruments C2000 Processors  SourceProductBaseCode=TIC2000
  wires:
  Data Store Read1/1 -> Digital Output1/1
  Data Store Read/1 -> Digital Output/1
  Data Store Read2/1 -> Digital Output2/1

== system TEST_IPM_2_0/INT/Current Sampling/First Order Filter  ==
  input : Inport
  Add : Sum  Inputs=+-
  Add3 : Sum  AccumDataTypeStr=single
  Constant : Constant  OutDataTypeStr=single  SampleTime=-1
  Data Store Read : DataStoreRead  DataStoreName=Udc_Filter
  Data Store Read2 : DataStoreRead  DataStoreName=Udc_Filter
  Gain : Gain  Gain=2*pi*Ts_10kHz
  Gain1 : Gain  Gain=2*pi*Ts_10kHz
  Product : Product
  Product1 : Product
  Unit Delay3 : UnitDelay  SampleTime=-1  HasFrameUpgradeWarning=on
  "output " : Outport
  wires:
  input/1 -> Product/1
  Product/1 -> Add3/1
  Product1/1 -> Unit Delay3/1
  Add3/1 -> Product1/1, "output "/1
  Unit Delay3/1 -> Add3/2
  Gain/1 -> Product/2
  Add/1 -> Product1/2
  Gain1/1 -> Add/2
  Constant/1 -> Add/1
  Data Store Read/1 -> Gain/1
  Data Store Read2/1 -> Gain1/1

== system TEST_IPM_2_0/INT/Extra Observer/Park Transformation ==
  Alpha : Inport
  Beta : Inport  Port=2
  theta : Inport  Port=3
  Add : Sum
  Add1 : Sum  Inputs=+-
  Gain : Gain  Gain=2*pi
  Product{,1..3} (4 alike) : Product
  Sin : Trigonometry  OutputSignalType=real
  Sin1 : Trigonometry  Operator=cos  OutputSignalType=real
  D : Outport
  Q : Outport  Port=2
  wires:
  Product/1 -> Add/1
  Sin/1 -> Product3/2, Product1/2
  Product1/1 -> Add/2
  Add1/1 -> Q/1
  Sin1/1 -> Product2/2, Product/2
  Product2/1 -> Add1/1
  Alpha/1 -> Product3/1, Product/1
  Beta/1 -> Product2/1, Product1/1
  Product3/1 -> Add1/2
  Add/1 -> D/1
  theta/1 -> Gain/1
  Gain/1 -> Sin/1, Sin1/1

== system TEST_IPM_2_0/INT/Extra Observer/Park Transformation1 ==
  Alpha : Inport
  Beta : Inport  Port=2
  theta : Inport  Port=3
  Add : Sum
  Add1 : Sum  Inputs=+-
  Gain : Gain  Gain=2*pi
  Product{,1..3} (4 alike) : Product
  Sin : Trigonometry  OutputSignalType=real
  Sin1 : Trigonometry  Operator=cos  OutputSignalType=real
  D : Outport
  Q : Outport  Port=2
  wires:
  Gain/1 -> Sin1/1, Sin/1
  theta/1 -> Gain/1
  Add/1 -> D/1
  Product3/1 -> Add1/2
  Beta/1 -> Product1/1, Product2/1
  Alpha/1 -> Product/1, Product3/1
  Product2/1 -> Add1/1
  Sin1/1 -> Product/2, Product2/2
  Add1/1 -> Q/1
  Product1/1 -> Add/2
  Sin/1 -> Product1/2, Product3/2
  Product/1 -> Add/1

== system TEST_IPM_2_0/INT/MAX5742/Subsystem ==
  function : TriggerPort  TriggerType=function-call  VariantControl=Variant
  Abs : Abs
  Add : Sum  Commented=on
  Add1 : Sum
  Add2 : Sum  Commented=on
  Add3 : Sum  Commented=on
  Add4 : Sum
  Constant : Constant  Commented=on  Value=100  OutDataTypeStr=single  SampleTime=-1
  Constant1 : Constant  Commented=on  Value=hex2dec('0000')  OutDataTypeStr=uint16  SampleTime=-1
  Constant2 : Constant  Value=hex2dec('0000')  OutDataTypeStr=uint16  SampleTime=-1
  Constant3 : Constant  Commented=on  Value=hex2dec('0000')  OutDataTypeStr=uint16  SampleTime=-1
  Constant4 : Constant  Value=30  OutDataTypeStr=single
  Data Store Read : DataStoreRead  Commented=on  DataStoreName=Id_FBK
  Data Store Read13 : DataStoreRead  DataStoreName=Id_FBK
  Data Store Read36 : DataStoreRead  Commented=on  DataStoreName=DEKF_Rs
  Gain : Gain  Commented=on  Gain=1/300*4095
  Gain1 : Gain  Commented=on  Gain=1/100*4095
  Gain2 : Gain  Gain=1/500*4095
  SPI Transmit : c280xlib/SPI Transmit  Commented=on  SPISelect=SPI_B  ClockPolarity=Rising_edge  ClockPhase=No_delay  SPIModule=uint32(0)  Mode=Master  BusSpeed=uint32(1000000)  FirstBitToTransfer=Most significant bit (MSB)  ClockMode=0  BlockFunction=Write  EnableRegisterAddress=on  RegisterAddress=0  OutputDataType=int8  OutputDataLength=1  BlockingMode=off  DataBits=16  UseCustomSSPin=Provided by the SPI peripheral  ActiveLowSSPin=Active low  Pin=0
      settings: SourceProductName=Embedded Coder Support Package for Texas Instruments C2000 Processors  SourceProductBaseCode=TIC2000
  SPI Transmit1 : c280xlib/SPI Transmit  Commented=on  SPISelect=SPI_B  ClockPolarity=Rising_edge  ClockPhase=No_delay  SPIModule=uint32(0)  Mode=Master  BusSpeed=uint32(1000000)  FirstBitToTransfer=Most significant bit (MSB)  ClockMode=0  BlockFunction=Write  EnableRegisterAddress=on  RegisterAddress=0  OutputDataType=int8  OutputDataLength=1  BlockingMode=off  DataBits=16  UseCustomSSPin=Provided by the SPI peripheral  ActiveLowSSPin=Active low  Pin=0
      settings: SourceProductName=Embedded Coder Support Package for Texas Instruments C2000 Processors  SourceProductBaseCode=TIC2000
  SPI Transmit2 : c280xlib/SPI Transmit  SPISelect=SPI_B  ClockPolarity=Rising_edge  ClockPhase=No_delay  SPIModule=uint32(0)  Mode=Master  BusSpeed=uint32(1000000)  FirstBitToTransfer=Most significant bit (MSB)  ClockMode=0  BlockFunction=Write  EnableRegisterAddress=on  RegisterAddress=0  OutputDataType=int8  OutputDataLength=1  BlockingMode=off  DataBits=16  UseCustomSSPin=Provided by the SPI peripheral  ActiveLowSSPin=Active low  Pin=0
      settings: SourceProductName=Embedded Coder Support Package for Texas Instruments C2000 Processors  SourceProductBaseCode=TIC2000
  Saturation : Saturate  Commented=on  UpperLimit=4095  LowerLimit=0  OutDataTypeStr=uint16
  Saturation1 : Saturate  Commented=on  UpperLimit=4095  LowerLimit=0  OutDataTypeStr=uint16
  Saturation2 : Saturate  UpperLimit=4095  LowerLimit=0  OutDataTypeStr=uint16
  Terminator : Terminator  Commented=on
  Terminator1 : Terminator  Commented=on
  Terminator2 : Terminator
  wires:
  Constant1/1 -> Add2/2
  SPI Transmit/1 -> Terminator/1
  Saturation/1 -> Add2/1
  Add2/1 -> SPI Transmit/1
  Gain/1 -> Saturation/1
  Add/1 -> Gain/1
  Data Store Read/1 -> Add/1
  Constant/1 -> Add/2
  Add3/1 -> SPI Transmit1/1
  Data Store Read36/1 -> Gain1/1
  Saturation1/1 -> Add3/1
  SPI Transmit1/1 -> Terminator1/1
  Constant3/1 -> Add3/2
  Gain1/1 -> Saturation1/1
  Add1/1 -> SPI Transmit2/1
  Gain2/1 -> Saturation2/1
  Constant2/1 -> Add1/2
  SPI Transmit2/1 -> Terminator2/1
  Saturation2/1 -> Add1/1
  Abs/1 -> Gain2/1
  Constant4/1 -> Add4/2
  Add4/1 -> Abs/1
  Data Store Read13/1 -> Add4/1

== system TEST_IPM_2_0/INT/MAX5742/Subsystem1 ==
  function : TriggerPort  TriggerType=function-call  VariantControl=Variant
  Abs : Abs
  Add1 : Sum  Commented=on
  Add2 : Sum  Commented=on
  Add3 : Sum
  Constant1 : Constant  Commented=on  Value=hex2dec('1000')  OutDataTypeStr=uint16  SampleTime=-1
  Constant2 : Constant  Commented=on  Value=hex2dec('1000')  OutDataTypeStr=uint16  SampleTime=-1
  Constant3 : Constant  Value=hex2dec('1000')  OutDataTypeStr=uint16  SampleTime=-1
  Data Store Read1 : DataStoreRead  Commented=on  DataStoreName=Iq_FBK
  Data Store Read14 : DataStoreRead  DataStoreName=Iq_FBK
  Data Store Read37 : DataStoreRead  Commented=on  DataStoreName=DEKF_Ldd
  Gain1 : Gain  Commented=on  Gain=1/300*4095
  Gain2 : Gain  Commented=on  Gain=1/500*4095
  Gain3 : Gain  Gain=1/60*4095
  SPI Transmit1 : c280xlib/SPI Transmit  Commented=on  SPISelect=SPI_B  ClockPolarity=Rising_edge  ClockPhase=No_delay  SPIModule=uint32(0)  Mode=Master  BusSpeed=uint32(1000000)  FirstBitToTransfer=Most significant bit (MSB)  ClockMode=0  BlockFunction=Write  EnableRegisterAddress=on  RegisterAddress=0  OutputDataType=int8  OutputDataLength=1  BlockingMode=off  DataBits=16  UseCustomSSPin=Provided by the SPI peripheral  ActiveLowSSPin=Active low  Pin=0
      settings: SourceProductName=Embedded Coder Support Package for Texas Instruments C2000 Processors  SourceProductBaseCode=TIC2000
  SPI Transmit2 : c280xlib/SPI Transmit  Commented=on  SPISelect=SPI_B  ClockPolarity=Rising_edge  ClockPhase=No_delay  SPIModule=uint32(0)  Mode=Master  BusSpeed=uint32(1000000)  FirstBitToTransfer=Most significant bit (MSB)  ClockMode=0  BlockFunction=Write  EnableRegisterAddress=on  RegisterAddress=0  OutputDataType=int8  OutputDataLength=1  BlockingMode=off  DataBits=16  UseCustomSSPin=Provided by the SPI peripheral  ActiveLowSSPin=Active low  Pin=0
      settings: SourceProductName=Embedded Coder Support Package for Texas Instruments C2000 Processors  SourceProductBaseCode=TIC2000
  SPI Transmit3 : c280xlib/SPI Transmit  SPISelect=SPI_B  ClockPolarity=Rising_edge  ClockPhase=No_delay  SPIModule=uint32(0)  Mode=Master  BusSpeed=uint32(1000000)  FirstBitToTransfer=Most significant bit (MSB)  ClockMode=0  BlockFunction=Write  EnableRegisterAddress=on  RegisterAddress=0  OutputDataType=int8  OutputDataLength=1  BlockingMode=off  DataBits=16  UseCustomSSPin=Provided by the SPI peripheral  ActiveLowSSPin=Active low  Pin=0
      settings: SourceProductName=Embedded Coder Support Package for Texas Instruments C2000 Processors  SourceProductBaseCode=TIC2000
  Saturation1 : Saturate  Commented=on  UpperLimit=4095  LowerLimit=0  OutDataTypeStr=uint16
  Saturation2 : Saturate  Commented=on  UpperLimit=4095  LowerLimit=0  OutDataTypeStr=uint16
  Saturation3 : Saturate  UpperLimit=4095  LowerLimit=0  OutDataTypeStr=uint16
  Terminator1 : Terminator  Commented=on
  Terminator2 : Terminator  Commented=on
  Terminator3 : Terminator
  wires:
  Saturation1/1 -> Add1/1
  Add1/1 -> SPI Transmit1/1
  SPI Transmit1/1 -> Terminator1/1
  Constant2/1 -> Add1/2
  Data Store Read1/1 -> Gain1/1
  Gain1/1 -> Saturation1/1
  Saturation2/1 -> Add2/1
  Data Store Read37/1 -> Gain2/1
  Add2/1 -> SPI Transmit2/1
  Constant1/1 -> Add2/2
  SPI Transmit2/1 -> Terminator2/1
  Gain2/1 -> Saturation2/1
  Data Store Read14/1 -> Abs/1
  Constant3/1 -> Add3/2
  Gain3/1 -> Saturation3/1
  Saturation3/1 -> Add3/1
  SPI Transmit3/1 -> Terminator3/1
  Add3/1 -> SPI Transmit3/1
  Abs/1 -> Gain3/1

== system TEST_IPM_2_0/INT/MAX5742/Subsystem2 ==
  function : TriggerPort  TriggerType=function-call  VariantControl=Variant
  Abs : Abs  Commented=on  OutDataTypeStr=single
  Add1 : Sum  Commented=on
  Add2 : Sum
  Add4 : Sum  Commented=on
  Constant1 : Constant  Commented=on  Value=hex2dec('2000')  OutDataTypeStr=uint16  SampleTime=-1
  Constant2 : Constant  Value=hex2dec('2000')  OutDataTypeStr=uint16  SampleTime=-1
  Constant5 : Constant  Commented=on  Value=hex2dec('2000')  OutDataTypeStr=uint16  SampleTime=-1
  Data Store Read : DataStoreRead  Commented=on  DataStoreName=Tr_Ttotal
  Data Store Read1 : DataStoreRead  DataStoreName=N_FBK
  Data Store Read38 : DataStoreRead  Commented=on  DataStoreName=DEKF_Ldq
  Gain1 : Gain  Commented=on  Gain=1/100*4095
  Gain2 : Gain  Commented=on  Gain=1/200*4095
  Gain3 : Gain  Gain=1/2000*4095
  SPI Transmit1 : c280xlib/SPI Transmit  Commented=on  SPISelect=SPI_B  ClockPolarity=Rising_edge  ClockPhase=No_delay  SPIModule=uint32(0)  Mode=Master  BusSpeed=uint32(1000000)  FirstBitToTransfer=Most significant bit (MSB)  ClockMode=0  BlockFunction=Write  EnableRegisterAddress=on  RegisterAddress=0  OutputDataType=int8  OutputDataLength=1  BlockingMode=off  DataBits=16  UseCustomSSPin=Provided by the SPI peripheral  ActiveLowSSPin=Active low  Pin=0
      settings: SourceProductName=Embedded Coder Support Package for Texas Instruments C2000 Processors  SourceProductBaseCode=TIC2000
  SPI Transmit2 : c280xlib/SPI Transmit  Commented=on  SPISelect=SPI_B  ClockPolarity=Rising_edge  ClockPhase=No_delay  SPIModule=uint32(0)  Mode=Master  BusSpeed=uint32(1000000)  FirstBitToTransfer=Most significant bit (MSB)  ClockMode=0  BlockFunction=Write  EnableRegisterAddress=on  RegisterAddress=0  OutputDataType=int8  OutputDataLength=1  BlockingMode=off  DataBits=16  UseCustomSSPin=Provided by the SPI peripheral  ActiveLowSSPin=Active low  Pin=0
      settings: SourceProductName=Embedded Coder Support Package for Texas Instruments C2000 Processors  SourceProductBaseCode=TIC2000
  SPI Transmit3 : c280xlib/SPI Transmit  SPISelect=SPI_B  ClockPolarity=Rising_edge  ClockPhase=No_delay  SPIModule=uint32(0)  Mode=Master  BusSpeed=uint32(1000000)  FirstBitToTransfer=Most significant bit (MSB)  ClockMode=0  BlockFunction=Write  EnableRegisterAddress=on  RegisterAddress=0  OutputDataType=int8  OutputDataLength=1  BlockingMode=off  DataBits=16  UseCustomSSPin=Provided by the SPI peripheral  ActiveLowSSPin=Active low  Pin=0
      settings: SourceProductName=Embedded Coder Support Package for Texas Instruments C2000 Processors  SourceProductBaseCode=TIC2000
  Saturation1 : Saturate  Commented=on  UpperLimit=4095  LowerLimit=0  OutDataTypeStr=uint16
  Saturation2 : Saturate  Commented=on  UpperLimit=4095  LowerLimit=0  OutDataTypeStr=uint16
  Saturation3 : Saturate  UpperLimit=4095  LowerLimit=0  OutDataTypeStr=uint16
  Terminator1 : Terminator  Commented=on
  Terminator2 : Terminator  Commented=on
  Terminator3 : Terminator
  wires:
  Constant5/1 -> Add4/2
  Saturation2/1 -> Add4/1
  Add4/1 -> SPI Transmit2/1
  SPI Transmit2/1 -> Terminator2/1
  Gain2/1 -> Saturation2/1
  Data Store Read/1 -> Gain2/1
  Saturation1/1 -> Add1/1
  Constant1/1 -> Add1/2
  Data Store Read38/1 -> Abs/1
  SPI Transmit1/1 -> Terminator1/1
  Gain1/1 -> Saturation1/1
  Add1/1 -> SPI Transmit1/1
  Abs/1 -> Gain1/1
  Gain3/1 -> Saturation3/1
  Add2/1 -> SPI Transmit3/1
  Constant2/1 -> Add2/2
  Saturation3/1 -> Add2/1
  Data Store Read1/1 -> Gain3/1
  SPI Transmit3/1 -> Terminator3/1
